simulink model "questao1exp3"  (R2026a)
settings: Solver=VariableStepAuto  MaxStep=0.00001
settings Model: Creator=cayon  LastModifiedBy=cayon

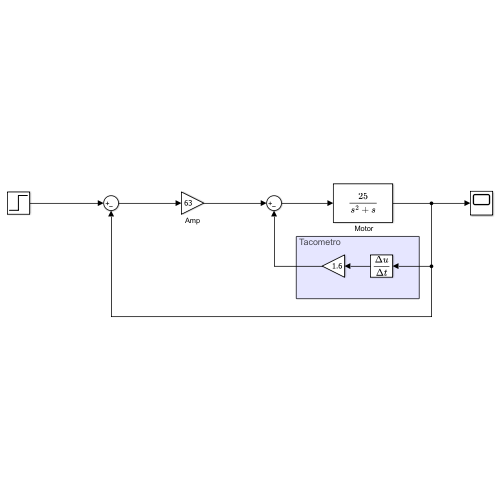
[thumbnail: Simulink's stored preview of the top-level diagram]
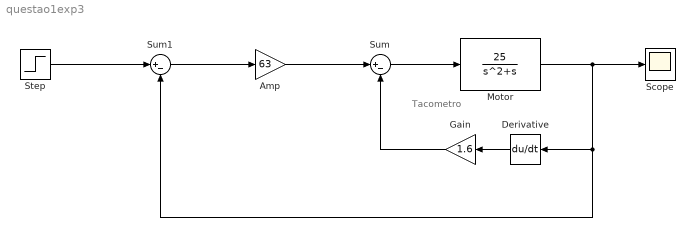
== system questao1exp3 ==
  note: Tacometro
  " Motor" : TransferFcn  Numerator=[25]  Denominator=[1 1 0]
  Amp : Gain  Gain=63
  Derivative : Derivative
  Gain : Gain  Gain=1.6
  Scope : Scope
      settings: ActiveDisplayYMinimum=0.015544288952093921  ActiveDisplayYMaximum=1.1984487644446635
  Step : Step  SampleTime=0
  Sum : Sum  Inputs=|+-
  Sum1 : Sum  Inputs=|+-
  wires:
  Derivative/1 -> Gain/1
  " Motor"/1 -> Sum1/2, Derivative/1, Scope/1
  Gain/1 -> Sum/2
  Amp/1 -> Sum/1
  Sum/1 -> " Motor"/1
  Sum1/1 -> Amp/1
  Step/1 -> Sum1/1
